simulink model "untitled1"  (R2021a)
settings: Solver=VariableStepAuto  StartTime=0.0  StopTime=10.0  RelTol=1e-3
undefined symbols (not defined in the file or in its folder): y
settings Model: Creator=surya  LastModifiedBy=surya

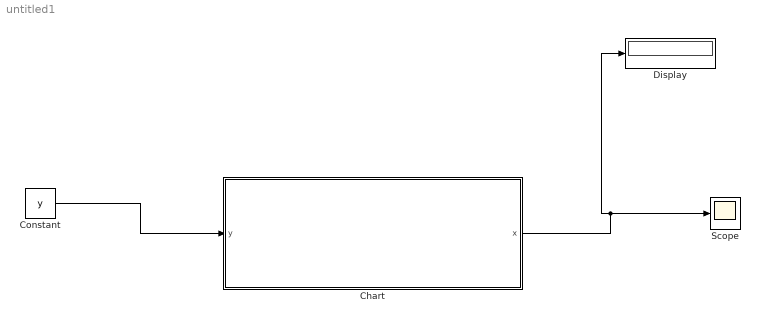
== system untitled1 ==
  Chart : Stateflow chart  TreatAsAtomicUnit=on
  Constant : Constant  Value=y
  Display : Display
  Scope : Scope
  wires:
  Constant/1 -> Chart/1(y)
  Chart/1(x) -> Scope/1, Display/1

== stateflow chart untitled1/Chart ==
  (default) -> (junction 21) : {t=0,out=y(1)}
  (junction 21) -> (junction 23)
  (junction 23) -> (junction 22) [order 1] : [t>=30]
  (junction 24) -> (junction 23)
  (junction 22) -> (junction 24) : {t=t+1;}
  (junction 23) -> (junction 25) [order 2]
  (junction 25) -> (junction 11)
  data: y input; x output
